simulink model "Geneva_Drive"  (R2015b)
settings: Solver=ode15s  StartTime=0.0  StopTime=30  MaxStep=1e-2  RelTol=1e-4  AbsTol=1e-5
PostLoadFcn:
  | set_param(bdroot,'IgnoredZcDiagnostic','none')
  | warning off sm:compiler:topologyAnalysis:DanglingBlock
StartFcn:
  | tic;
StopFcn:
  | Elapsed_Sim_Time = toc;
  | disp(['Elapsed Sim Time = ' num2str(Elapsed_Sim_Time)]);
undefined symbols (not defined in the file): X, Y, Z
libraries: sm_lib x44, Contact_Forces_Lib x20, nesl_utility x5, simulink x1
(part 2 of 2)

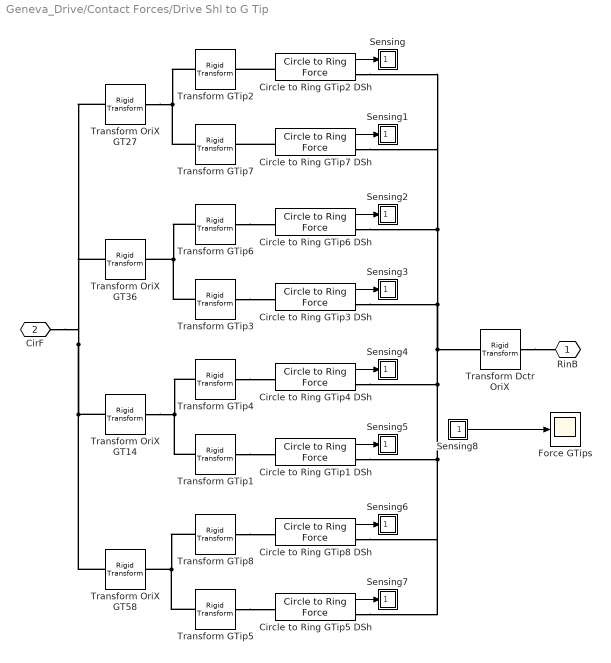
== system Geneva_Drive/Contact Forces/Drive Shl to G Tip ==
  Circle to Ring GTip1 DSh : Contact_Forces_Lib/2D/Circle to Ring Force  radius_circle=r_genv_cir  radius_ring=r_shld-d_shld/2  d_ring=d_shld  active_angle=[-90 180]  force_law=Linear  k_contact=k_contact  b_contact=b_contact  pen_full_damp_F=1e-4  pen_exponent=1  custom_param_1=1  custom_param_2=1  friction_law=None  mu_kinetic=0.5  mu_static=0.7  v_thr=0.001
  Circle to Ring GTip2 DSh : Contact_Forces_Lib/2D/Circle to Ring Force  radius_circle=r_genv_cir  radius_ring=r_shld-d_shld/2  d_ring=d_shld  active_angle=[-90 180]  force_law=Linear  k_contact=k_contact  b_contact=b_contact  pen_full_damp_F=1e-4  pen_exponent=1  custom_param_1=1  custom_param_2=1  friction_law=None  mu_kinetic=0.5  mu_static=0.7  v_thr=0.001
  Circle to Ring GTip3 DSh : Contact_Forces_Lib/2D/Circle to Ring Force  radius_circle=r_genv_cir  radius_ring=r_shld-d_shld/2  d_ring=d_shld  active_angle=[-90 180]  force_law=Linear  k_contact=k_contact  b_contact=b_contact  pen_full_damp_F=1e-4  pen_exponent=1  custom_param_1=1  custom_param_2=1  friction_law=None  mu_kinetic=0.5  mu_static=0.7  v_thr=0.001
  Circle to Ring GTip4 DSh : Contact_Forces_Lib/2D/Circle to Ring Force  radius_circle=r_genv_cir  radius_ring=r_shld-d_shld/2  d_ring=d_shld  active_angle=[-90 180]  force_law=Linear  k_contact=k_contact  b_contact=b_contact  pen_full_damp_F=1e-4  pen_exponent=1  custom_param_1=1  custom_param_2=1  friction_law=None  mu_kinetic=0.5  mu_static=0.7  v_thr=0.001
  Circle to Ring GTip5 DSh : Contact_Forces_Lib/2D/Circle to Ring Force  radius_circle=r_genv_cir  radius_ring=r_shld-d_shld/2  d_ring=d_shld  active_angle=[-90 180]  force_law=Linear  k_contact=k_contact  b_contact=b_contact  pen_full_damp_F=1e-4  pen_exponent=1  custom_param_1=1  custom_param_2=1  friction_law=None  mu_kinetic=0.5  mu_static=0.7  v_thr=0.001
  Circle to Ring GTip6 DSh : Contact_Forces_Lib/2D/Circle to Ring Force  radius_circle=r_genv_cir  radius_ring=r_shld-d_shld/2  d_ring=d_shld  active_angle=[-90 180]  force_law=Linear  k_contact=k_contact  b_contact=b_contact  pen_full_damp_F=1e-4  pen_exponent=1  custom_param_1=1  custom_param_2=1  friction_law=None  mu_kinetic=0.5  mu_static=0.7  v_thr=0.001
  Circle to Ring GTip7 DSh : Contact_Forces_Lib/2D/Circle to Ring Force  radius_circle=r_genv_cir  radius_ring=r_shld-d_shld/2  d_ring=d_shld  active_angle=[-90 180]  force_law=Linear  k_contact=k_contact  b_contact=b_contact  pen_full_damp_F=1e-4  pen_exponent=1  custom_param_1=1  custom_param_2=1  friction_law=None  mu_kinetic=0.5  mu_static=0.7  v_thr=0.001
  Circle to Ring GTip8 DSh : Contact_Forces_Lib/2D/Circle to Ring Force  radius_circle=r_genv_cir  radius_ring=r_shld-d_shld/2  d_ring=d_shld  active_angle=[-90 180]  force_law=Linear  k_contact=k_contact  b_contact=b_contact  pen_full_damp_F=1e-4  pen_exponent=1  custom_param_1=1  custom_param_2=1  friction_law=None  mu_kinetic=0.5  mu_static=0.7  v_thr=0.001
  Force GTips : Scope
  Sensing : Subsystem
  Sensing1 : Subsystem
  Sensing2 : Subsystem
  Sensing3 : Subsystem
  Sensing4 : Subsystem
  Sensing5 : Subsystem
  Sensing6 : Subsystem
  Sensing7 : Subsystem
  Sensing8 : Subsystem
  Transform Dctr OriX : sm_lib/Frames and Transforms/Rigid Transform  TranslationMethod=None  TranslationLengthUnit=m  TranslationStandardAxis=+Z  TranslationStandardOffset=0  TranslationCartesianOffset=[0 0 0]  TranslationROffset=0  TranslationROffsetUnits=m  TranslationZOffset=0  TranslationZOffsetUnits=m  TranslationThetaOffset=0  TranslationThetaOffsetUnits=deg  RotationMethod=AlignedAxes  RotationAngleUnits=deg  RotationStandardAxis=+Z  RotationAngle=180  RotationArbitraryAxis=[0 0 1]  FollAlignAxisA=+X  BaseAlignAxisA=-X  FollAlignAxisB=+Z  BaseAlignAxisB=-Z  RotationSequenceAxes=FollowerAxes  RotationSequence=XYX  RotationSequenceAngles=[0 0 0]  RotationSequenceAnglesUnits=deg  RotationMatrix=[1 0 0; 0 1 0; 0 0 1]  BlockFunction=simmechanics.library.frames_transforms.rigid_transform
  Transform GTip{1,3,5,7} (4 alike) : sm_lib/Frames and Transforms/Rigid Transform  TranslationMethod=Cartesian  TranslationLengthUnit=m  TranslationStandardAxis=+Y  TranslationStandardOffset=0.1405  TranslationCartesianOffset=[-0.022 -0.139 0]  TranslationROffset=0  TranslationROffsetUnits=m  TranslationZOffset=0  TranslationZOffsetUnits=m  TranslationThetaOffset=0  TranslationThetaOffsetUnits=deg  RotationMethod=None  RotationAngleUnits=deg  RotationStandardAxis=+Z  RotationAngle=45  RotationArbitraryAxis=[0 0 1]  FollAlignAxisA=+X  BaseAlignAxisA=+Y  FollAlignAxisB=+Y  BaseAlignAxisB=+Z  RotationSequenceAxes=FollowerAxes  RotationSequence=XYX  RotationSequenceAngles=[0 0 0]  RotationSequenceAnglesUnits=deg  RotationMatrix=[1 0 0; 0 1 0; 0 0 1]  BlockFunction=simmechanics.library.frames_transforms.rigid_transform
  Transform GTip{2,4,6,8} (4 alike) : sm_lib/Frames and Transforms/Rigid Transform  TranslationMethod=Cartesian  TranslationLengthUnit=m  TranslationStandardAxis=+Y  TranslationStandardOffset=0.1405  TranslationCartesianOffset=[-0.022 0.139 0]  TranslationROffset=0  TranslationROffsetUnits=m  TranslationZOffset=0  TranslationZOffsetUnits=m  TranslationThetaOffset=0  TranslationThetaOffsetUnits=deg  RotationMethod=None  RotationAngleUnits=deg  RotationStandardAxis=+Z  RotationAngle=45  RotationArbitraryAxis=[0 0 1]  FollAlignAxisA=+X  BaseAlignAxisA=+Y  FollAlignAxisB=+Y  BaseAlignAxisB=+Z  RotationSequenceAxes=FollowerAxes  RotationSequence=XYX  RotationSequenceAngles=[0 0 0]  RotationSequenceAnglesUnits=deg  RotationMatrix=[1 0 0; 0 1 0; 0 0 1]  BlockFunction=simmechanics.library.frames_transforms.rigid_transform
  Transform OriX GT14 : sm_lib/Frames and Transforms/Rigid Transform  TranslationMethod=None  TranslationLengthUnit=m  TranslationStandardAxis=+Z  TranslationStandardOffset=0  TranslationCartesianOffset=[0 0 0]  TranslationROffset=0  TranslationROffsetUnits=m  TranslationZOffset=0  TranslationZOffsetUnits=m  TranslationThetaOffset=0  TranslationThetaOffsetUnits=deg  RotationMethod=StandardAxis  RotationAngleUnits=deg  RotationStandardAxis=+Z  RotationAngle=225  RotationArbitraryAxis=[0 0 1]  FollAlignAxisA=+X  BaseAlignAxisA=+Y  FollAlignAxisB=+Y  BaseAlignAxisB=+Z  RotationSequenceAxes=FollowerAxes  RotationSequence=XYX  RotationSequenceAngles=[0 0 0]  RotationSequenceAnglesUnits=deg  RotationMatrix=[1 0 0; 0 1 0; 0 0 1]  BlockFunction=simmechanics.library.frames_transforms.rigid_transform
  Transform OriX GT27 : sm_lib/Frames and Transforms/Rigid Transform  TranslationMethod=None  TranslationLengthUnit=m  TranslationStandardAxis=+Z  TranslationStandardOffset=0  TranslationCartesianOffset=[0 0 0]  TranslationROffset=0  TranslationROffsetUnits=m  TranslationZOffset=0  TranslationZOffsetUnits=m  TranslationThetaOffset=0  TranslationThetaOffsetUnits=deg  RotationMethod=StandardAxis  RotationAngleUnits=deg  RotationStandardAxis=+Z  RotationAngle=315  RotationArbitraryAxis=[0 0 1]  FollAlignAxisA=+X  BaseAlignAxisA=+Y  FollAlignAxisB=+Y  BaseAlignAxisB=+Z  RotationSequenceAxes=FollowerAxes  RotationSequence=XYX  RotationSequenceAngles=[0 0 0]  RotationSequenceAnglesUnits=deg  RotationMatrix=[1 0 0; 0 1 0; 0 0 1]  BlockFunction=simmechanics.library.frames_transforms.rigid_transform
  Transform OriX GT36 : sm_lib/Frames and Transforms/Rigid Transform  TranslationMethod=None  TranslationLengthUnit=m  TranslationStandardAxis=+Z  TranslationStandardOffset=0  TranslationCartesianOffset=[0 0 0]  TranslationROffset=0  TranslationROffsetUnits=m  TranslationZOffset=0  TranslationZOffsetUnits=m  TranslationThetaOffset=0  TranslationThetaOffsetUnits=deg  RotationMethod=StandardAxis  RotationAngleUnits=deg  RotationStandardAxis=+Z  RotationAngle=135  RotationArbitraryAxis=[0 0 1]  FollAlignAxisA=+X  BaseAlignAxisA=+Y  FollAlignAxisB=+Y  BaseAlignAxisB=+Z  RotationSequenceAxes=FollowerAxes  RotationSequence=XYX  RotationSequenceAngles=[0 0 0]  RotationSequenceAnglesUnits=deg  RotationMatrix=[1 0 0; 0 1 0; 0 0 1]  BlockFunction=simmechanics.library.frames_transforms.rigid_transform
  Transform OriX GT58 : sm_lib/Frames and Transforms/Rigid Transform  TranslationMethod=None  TranslationLengthUnit=m  TranslationStandardAxis=+Z  TranslationStandardOffset=0  TranslationCartesianOffset=[0 0 0]  TranslationROffset=0  TranslationROffsetUnits=m  TranslationZOffset=0  TranslationZOffsetUnits=m  TranslationThetaOffset=0  TranslationThetaOffsetUnits=deg  RotationMethod=StandardAxis  RotationAngleUnits=deg  RotationStandardAxis=+Z  RotationAngle=45  RotationArbitraryAxis=[0 0 1]  FollAlignAxisA=+X  BaseAlignAxisA=+Y  FollAlignAxisB=+Y  BaseAlignAxisB=+Z  RotationSequenceAxes=FollowerAxes  RotationSequence=XYX  RotationSequenceAngles=[0 0 0]  RotationSequenceAnglesUnits=deg  RotationMatrix=[1 0 0; 0 1 0; 0 0 1]  BlockFunction=simmechanics.library.frames_transforms.rigid_transform
  RinB : PMIOPort  Port=1  Side=Right
  CirF : PMIOPort  Port=2  Side=Left
  wires:
  Sensing8/1(S) -> Force GTips/1
  Circle to Ring GTip5 DSh/1 -> Sensing7/1(S)
  Circle to Ring GTip8 DSh/1 -> Sensing6/1(S)
  Circle to Ring GTip2 DSh/1 -> Sensing/1(S)
  Circle to Ring GTip6 DSh/1 -> Sensing2/1(S)
  Circle to Ring GTip4 DSh/1 -> Sensing4/1(S)
  Circle to Ring GTip7 DSh/1 -> Sensing1/1(S)
  Circle to Ring GTip3 DSh/1 -> Sensing3/1(S)
  Circle to Ring GTip1 DSh/1 -> Sensing5/1(S)
  connections:
  Transform GTip8/LConn1 -- Transform GTip5/LConn1 -- Transform OriX GT58/RConn1
  Transform GTip5/RConn1 -- Circle to Ring GTip5 DSh/LConn1
  Circle to Ring GTip3 DSh/RConn1 -- Transform Dctr OriX/RConn1 -- Circle to Ring GTip4 DSh/RConn1 -- Circle to Ring GTip1 DSh/RConn1 -- Circle to Ring GTip8 DSh/RConn1 -- Circle to Ring GTip5 DSh/RConn1 -- Circle to Ring GTip7 DSh/RConn1 -- Circle to Ring GTip2 DSh/RConn1 -- Circle to Ring GTip6 DSh/RConn1
  Transform GTip6/RConn1 -- Circle to Ring GTip6 DSh/LConn1
  Circle to Ring GTip7 DSh/LConn1 -- Transform GTip7/RConn1
  Circle to Ring GTip2 DSh/LConn1 -- Transform GTip2/RConn1
  Transform GTip8/RConn1 -- Circle to Ring GTip8 DSh/LConn1
  Transform GTip1/RConn1 -- Circle to Ring GTip1 DSh/LConn1
  Transform GTip4/RConn1 -- Circle to Ring GTip4 DSh/LConn1
  Transform GTip3/RConn1 -- Circle to Ring GTip3 DSh/LConn1
  Transform OriX GT27/RConn1 -- Transform GTip2/LConn1 -- Transform GTip7/LConn1
  Transform GTip3/LConn1 -- Transform GTip6/LConn1 -- Transform OriX GT36/RConn1
  Transform OriX GT14/LConn1 -- Transform OriX GT58/LConn1 -- Transform OriX GT36/LConn1 -- Transform OriX GT27/LConn1 -- CirF/RConn1
  Transform GTip1/LConn1 -- Transform GTip4/LConn1 -- Transform OriX GT14/RConn1
  Transform Dctr OriX/LConn1 -- RinB/RConn1

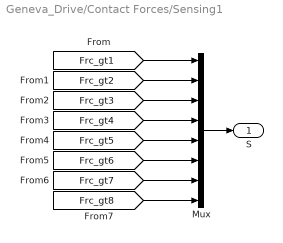
== system Geneva_Drive/Contact Forces/Sensing1 ==
  Mux : Mux  Inputs=8
  S : Outport
  wires:
  [Frc_gt6] -> Mux/6
  [Frc_gt5] -> Mux/5
  [Frc_gt8] -> Mux/8
  [Frc_gt7] -> Mux/7
  [Frc_gt4] -> Mux/4
  [Frc_gt2] -> Mux/2
  [Frc_gt3] -> Mux/3
  [Frc_gt1] -> Mux/1
  Mux/1 -> S/1

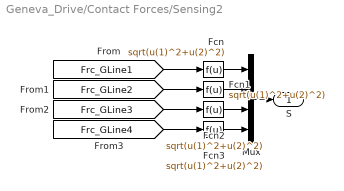
== system Geneva_Drive/Contact Forces/Sensing2 ==
  Fcn{,1..3} (4 alike) : Fcn  Expr=sqrt(u(1)^2+u(2)^2)
  Mux : Mux
  S : Outport
  wires:
  Fcn3/1 -> Mux/4
  Fcn2/1 -> Mux/3
  Fcn1/1 -> Mux/2
  Fcn/1 -> Mux/1
  [Frc_GLine4] -> Fcn3/1
  [Frc_GLine2] -> Fcn1/1
  [Frc_GLine3] -> Fcn2/1
  [Frc_GLine1] -> Fcn/1
  Mux/1 -> S/1

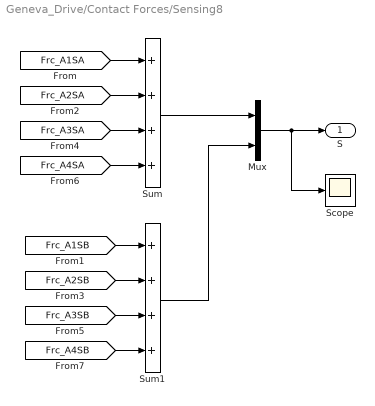
== system Geneva_Drive/Contact Forces/Sensing8 ==
  Mux : Mux  Inputs=2
  Scope : Scope
  Sum : Sum  Inputs=++++
  Sum1 : Sum  Inputs=++++
  S : Outport
  wires:
  Sum1/1 -> Mux/2
  Sum/1 -> Mux/1
  [Frc_A3SB] -> Sum1/3
  [Frc_A2SB] -> Sum1/2
  [Frc_A4SB] -> Sum1/4
  [Frc_A1SB] -> Sum1/1
  [Frc_A1SA] -> Sum/1
  [Frc_A4SA] -> Sum/4
  [Frc_A2SA] -> Sum/2
  [Frc_A3SA] -> Sum/3
  Mux/1 -> S/1, Scope/1

== system Geneva_Drive/Contact Forces/Drive Pin to G Slots/Sensing1 ==
  S : Inport
  Bus Selector : BusSelector  OutputSignals=FCir.Fx,FCir.Fy  OutputAsBus=on
  tag scope: Frc_GLine2=global
  wires:
  S/1 -> Bus Selector/1
  Bus Selector/1 -> [Frc_GLine2]

== system Geneva_Drive/Contact Forces/Drive Pin to G Slots/Sensing2 ==
  S : Inport
  Bus Selector : BusSelector  OutputSignals=FCir.Fx,FCir.Fy  OutputAsBus=on
  tag scope: Frc_GLine3=global
  wires:
  S/1 -> Bus Selector/1
  Bus Selector/1 -> [Frc_GLine3]

== system Geneva_Drive/Contact Forces/Drive Pin to G Slots/Sensing3 ==
  S : Inport
  Bus Selector : BusSelector  OutputSignals=FCir.Fx,FCir.Fy  OutputAsBus=on
  tag scope: Frc_GLine1=global
  wires:
  S/1 -> Bus Selector/1
  Bus Selector/1 -> [Frc_GLine1]

== system Geneva_Drive/Contact Forces/Drive Pin to G Slots/Sensing4 ==
  S : Inport
  Bus Selector : BusSelector  OutputSignals=FCir.Fx,FCir.Fy  OutputAsBus=on
  tag scope: Frc_GLine4=global
  wires:
  S/1 -> Bus Selector/1
  Bus Selector/1 -> [Frc_GLine4]

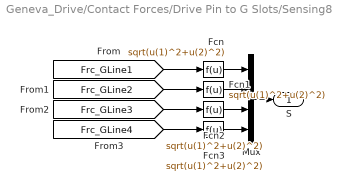
== system Geneva_Drive/Contact Forces/Drive Pin to G Slots/Sensing8 ==
  Fcn{,1..3} (4 alike) : Fcn  Expr=sqrt(u(1)^2+u(2)^2)
  Mux : Mux
  S : Outport
  wires:
  Fcn3/1 -> Mux/4
  Fcn2/1 -> Mux/3
  Fcn1/1 -> Mux/2
  Fcn/1 -> Mux/1
  [Frc_GLine4] -> Fcn3/1
  [Frc_GLine2] -> Fcn1/1
  [Frc_GLine3] -> Fcn2/1
  [Frc_GLine1] -> Fcn/1
  Mux/1 -> S/1

== system Geneva_Drive/Contact Forces/Drive Shl to G Arc/Sensing ==
  S : Inport
  Bus Selector : BusSelector  OutputSignals=Normal Force
  tag scope: Frc_A2SA=global
  wires:
  S/1 -> Bus Selector/1
  Bus Selector/1 -> [Frc_A2SA]  "<Normal Force>"

== system Geneva_Drive/Contact Forces/Drive Shl to G Arc/Sensing1 ==
  S : Inport
  Bus Selector : BusSelector  OutputSignals=Normal Force
  tag scope: Frc_A2SB=global
  wires:
  S/1 -> Bus Selector/1
  Bus Selector/1 -> [Frc_A2SB]  "<Normal Force>"

== system Geneva_Drive/Contact Forces/Drive Shl to G Arc/Sensing2 ==
  S : Inport
  Bus Selector : BusSelector  OutputSignals=Normal Force
  tag scope: Frc_A3SA=global
  wires:
  S/1 -> Bus Selector/1
  Bus Selector/1 -> [Frc_A3SA]  "<Normal Force>"

== system Geneva_Drive/Contact Forces/Drive Shl to G Arc/Sensing3 ==
  S : Inport
  Bus Selector : BusSelector  OutputSignals=Normal Force
  tag scope: Frc_A3SB=global
  wires:
  S/1 -> Bus Selector/1
  Bus Selector/1 -> [Frc_A3SB]  "<Normal Force>"

== system Geneva_Drive/Contact Forces/Drive Shl to G Arc/Sensing4 ==
  S : Inport
  Bus Selector : BusSelector  OutputSignals=Normal Force
  tag scope: Frc_A4SA=global
  wires:
  S/1 -> Bus Selector/1
  Bus Selector/1 -> [Frc_A4SA]  "<Normal Force>"

== system Geneva_Drive/Contact Forces/Drive Shl to G Arc/Sensing5 ==
  S : Inport
  Bus Selector : BusSelector  OutputSignals=Normal Force
  tag scope: Frc_A4SB=global
  wires:
  S/1 -> Bus Selector/1
  Bus Selector/1 -> [Frc_A4SB]  "<Normal Force>"

== system Geneva_Drive/Contact Forces/Drive Shl to G Arc/Sensing6 ==
  S : Inport
  Bus Selector : BusSelector  OutputSignals=Normal Force
  tag scope: Frc_A1SA=global
  wires:
  S/1 -> Bus Selector/1
  Bus Selector/1 -> [Frc_A1SA]  "<Normal Force>"

== system Geneva_Drive/Contact Forces/Drive Shl to G Arc/Sensing7 ==
  S : Inport
  Bus Selector : BusSelector  OutputSignals=Normal Force
  tag scope: Frc_A1SB=global
  wires:
  S/1 -> Bus Selector/1
  Bus Selector/1 -> [Frc_A1SB]  "<Normal Force>"

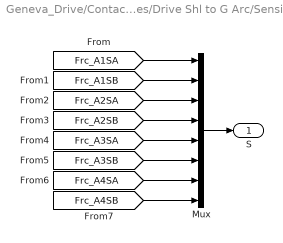
== system Geneva_Drive/Contact Forces/Drive Shl to G Arc/Sensing8 ==
  Mux : Mux  Inputs=8
  S : Outport
  wires:
  [Frc_A3SB] -> Mux/6
  [Frc_A3SA] -> Mux/5
  [Frc_A4SB] -> Mux/8
  [Frc_A4SA] -> Mux/7
  [Frc_A2SB] -> Mux/4
  [Frc_A1SB] -> Mux/2
  [Frc_A2SA] -> Mux/3
  [Frc_A1SA] -> Mux/1
  Mux/1 -> S/1

== system Geneva_Drive/Contact Forces/Drive Shl to G Tip/Sensing ==
  S : Inport
  Bus Selector : BusSelector  OutputSignals=Normal Force
  tag scope: Frc_gt2=global
  wires:
  S/1 -> Bus Selector/1
  Bus Selector/1 -> [Frc_gt2]  "<Normal Force>"

== system Geneva_Drive/Contact Forces/Drive Shl to G Tip/Sensing1 ==
  S : Inport
  Bus Selector : BusSelector  OutputSignals=Normal Force
  tag scope: Frc_gt7=global
  wires:
  S/1 -> Bus Selector/1
  Bus Selector/1 -> [Frc_gt7]  "<Normal Force>"

== system Geneva_Drive/Contact Forces/Drive Shl to G Tip/Sensing2 ==
  S : Inport
  Bus Selector : BusSelector  OutputSignals=Normal Force
  tag scope: Frc_gt6=global
  wires:
  S/1 -> Bus Selector/1
  Bus Selector/1 -> [Frc_gt6]  "<Normal Force>"

== system Geneva_Drive/Contact Forces/Drive Shl to G Tip/Sensing3 ==
  S : Inport
  Bus Selector : BusSelector  OutputSignals=Normal Force
  tag scope: Frc_gt3=global
  wires:
  S/1 -> Bus Selector/1
  Bus Selector/1 -> [Frc_gt3]  "<Normal Force>"

== system Geneva_Drive/Contact Forces/Drive Shl to G Tip/Sensing4 ==
  S : Inport
  Bus Selector : BusSelector  OutputSignals=Normal Force
  tag scope: Frc_gt4=global
  wires:
  S/1 -> Bus Selector/1
  Bus Selector/1 -> [Frc_gt4]  "<Normal Force>"

== system Geneva_Drive/Contact Forces/Drive Shl to G Tip/Sensing5 ==
  S : Inport
  Bus Selector : BusSelector  OutputSignals=Normal Force
  tag scope: Frc_gt1=global
  wires:
  S/1 -> Bus Selector/1
  Bus Selector/1 -> [Frc_gt1]  "<Normal Force>"

== system Geneva_Drive/Contact Forces/Drive Shl to G Tip/Sensing6 ==
  S : Inport
  Bus Selector : BusSelector  OutputSignals=Normal Force
  tag scope: Frc_gt8=global
  wires:
  S/1 -> Bus Selector/1
  Bus Selector/1 -> [Frc_gt8]  "<Normal Force>"

== system Geneva_Drive/Contact Forces/Drive Shl to G Tip/Sensing7 ==
  S : Inport
  Bus Selector : BusSelector  OutputSignals=Normal Force
  tag scope: Frc_gt5=global
  wires:
  S/1 -> Bus Selector/1
  Bus Selector/1 -> [Frc_gt5]  "<Normal Force>"

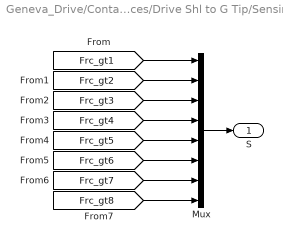
== system Geneva_Drive/Contact Forces/Drive Shl to G Tip/Sensing8 ==
  Mux : Mux  Inputs=8
  S : Outport
  wires:
  [Frc_gt6] -> Mux/6
  [Frc_gt5] -> Mux/5
  [Frc_gt8] -> Mux/8
  [Frc_gt7] -> Mux/7
  [Frc_gt4] -> Mux/4
  [Frc_gt2] -> Mux/2
  [Frc_gt3] -> Mux/3
  [Frc_gt1] -> Mux/1
  Mux/1 -> S/1
